simulink model "test"  (R2021b)
settings: Solver=FixedStepDiscrete  StartTime=0.0  StopTime=inf  RelTol=1e-3
settings Model: Creator=ACH  LastModifiedBy=angel
settings SolverCC: ConcurrentTasks=on  PositivePriorityOrder=on
settings OptimizationCC: BlockReduction=off  OptimizeBlockIOStorage=off
settings DebuggingCC: TasksWithSamePriorityMsg=none
settings HardwareCC: ProdBitPerLong=64  ProdLongLongMode=on  ProdHWDeviceType=Intel->x86-64 (Linux 64)
settings RTWCC: Description=Simulink Real-Time  SystemTargetFile=slrealtime.tlc  TemplateMakefile=slrealtime_default_tmf  Toolchain=Simulink Real-Time Toolchain  BuildConfiguration=Faster Runs  CodeExecutionProfiling=on  TargetLang=C++
settings SimulinkRealTimeTargetCC: UseGCCFastMath=on

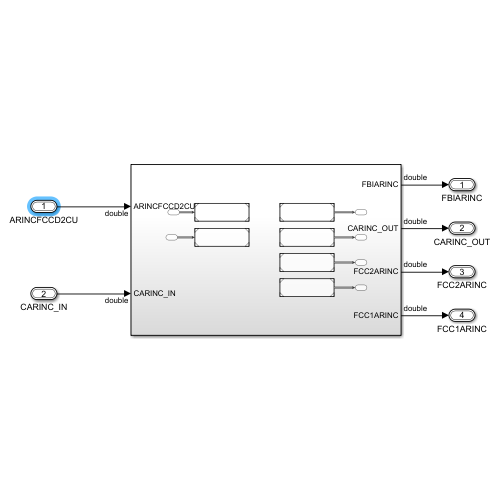
[thumbnail: Simulink's stored preview of the top-level diagram]
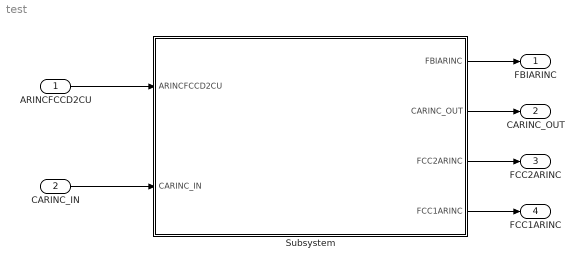
== system test ==
  ARINCFCCD2CU : Inport  OutDataTypeStr=Bus: ACE8C_FCC1
  CARINC_IN : Inport  Port=2  OutDataTypeStr=Bus: ACE9C_ACE8x_9C
  Subsystem : Subsystem
  FBIARINC : Outport  OutDataTypeStr=Bus: FBI_ACExxxA_C_A
  CARINC_OUT : Outport  Port=2  OutDataTypeStr=Bus: ACE9C_ACE8x_9C
  FCC2ARINC : Outport  Port=3  OutDataTypeStr=Bus: FCC2_ACExxxA_M_A
  FCC1ARINC : Outport  Port=4  OutDataTypeStr=Bus: FCC1_ACExxxA_C1_A
  wires:
  ARINCFCCD2CU/1 -> Subsystem/1(ARINCFCCD2CU)
  CARINC_IN/1 -> Subsystem/2(CARINC_IN)
  Subsystem/1(FBIARINC) -> FBIARINC/1
  Subsystem/2(CARINC_OUT) -> CARINC_OUT/1
  Subsystem/3(FCC2ARINC) -> FCC2ARINC/1
  Subsystem/4(FCC1ARINC) -> FCC1ARINC/1

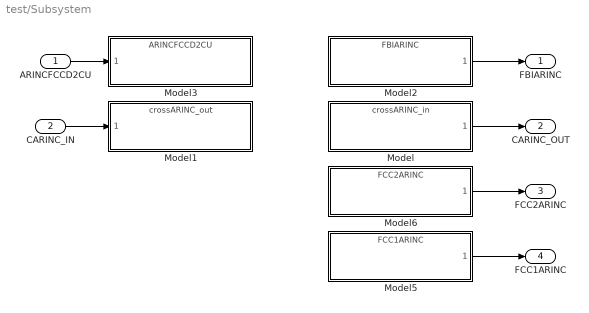
== system test/Subsystem ==
  ARINCFCCD2CU : Inport  OutDataTypeStr=Bus: ACE8C_FCC1
  CARINC_IN : Inport  Port=2  OutDataTypeStr=Bus: ACE9C_ACE8x_9C
  Model : ModelReference  ModelNameDialog=crossARINC_in.slx  SimulationMode=Normal  ModelReferenceVersion=1.30
  Model1 : ModelReference  ModelNameDialog=crossARINC_out.slx  SimulationMode=Normal  ModelReferenceVersion=1.48
  Model2 : ModelReference  ModelNameDialog=FBIARINC.slx  SimulationMode=Normal  ModelReferenceVersion=1.37
  Model3 : ModelReference  ModelNameDialog=ARINCFCCD2CU.slx  SimulationMode=Normal  ModelReferenceVersion=1.40
  Model5 : ModelReference  ModelNameDialog=FCC1ARINC.slx  SimulationMode=Normal  ModelReferenceVersion=1.41
  Model6 : ModelReference  ModelNameDialog=FCC2ARINC.slx  SimulationMode=Normal  ModelReferenceVersion=1.36
  FBIARINC : Outport  OutDataTypeStr=Bus: FBI_ACExxxA_C_A
  CARINC_OUT : Outport  Port=2  OutDataTypeStr=Bus: ACE9C_ACE8x_9C
  FCC2ARINC : Outport  Port=3  OutDataTypeStr=Bus: FCC2_ACExxxA_M_A
  FCC1ARINC : Outport  Port=4  OutDataTypeStr=Bus: FCC1_ACExxxA_C1_A
  wires:
  CARINC_IN/1 -> Model1/1
  Model/1 -> CARINC_OUT/1
  ARINCFCCD2CU/1 -> Model3/1
  Model5/1 -> FCC1ARINC/1
  Model2/1 -> FBIARINC/1
  Model6/1 -> FCC2ARINC/1
